simulink model "sampleModel646original"  (R2021b)
settings: Solver=VariableStepAuto  StartTime=0.0  StopTime=10.0  RelTol=1e-3
undefined symbols (not defined in the file): DiscIntNeverNeededParam, Newton, Raphson, sigbuilder_block
libraries: simulink x194, slpidlib x27
(part 1 of 5)
settings Model: Creator=user  LastModifiedBy=cemery

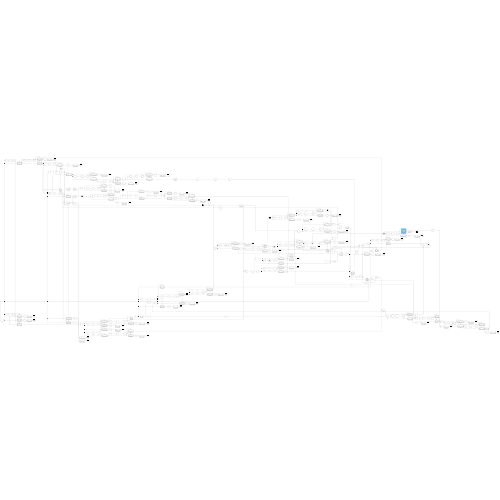
[thumbnail: Simulink's stored preview of the top-level diagram]
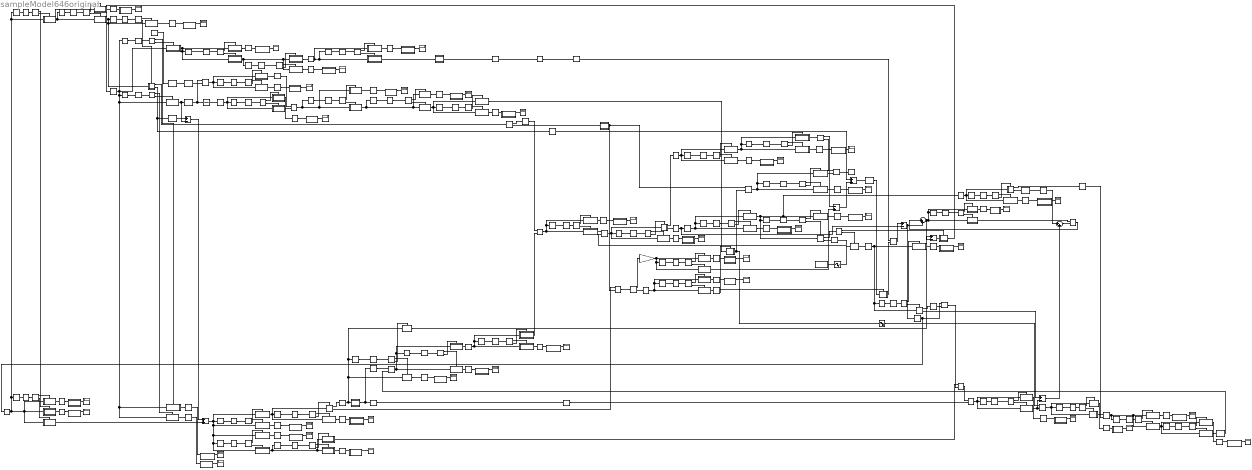
== system sampleModel646original ==
  cfblk1 : Delay  DelayLengthSource=Input port  SampleTime=1
      settings: InputPortMap=u0,p1
  cfblk10 : Subsystem  TreatAsAtomicUnit=on
  cfblk100 : Subsystem  TreatAsAtomicUnit=on
  cfblk101 : Subsystem  TreatAsAtomicUnit=on
  cfblk102 : Subsystem  TreatAsAtomicUnit=on
  cfblk{103..104,109..113} (7 alike) : Delay  SampleTime=1
  cfblk105 : Subsystem  TreatAsAtomicUnit=on
  cfblk106 : Subsystem  TreatAsAtomicUnit=on
  cfblk107 : Subsystem  TreatAsAtomicUnit=on
  cfblk108 : Subsystem  TreatAsAtomicUnit=on
  cfblk11 : Subsystem  TreatAsAtomicUnit=on
  cfblk12 : Subsystem  TreatAsAtomicUnit=on
  cfblk13 : Subsystem  TreatAsAtomicUnit=on
  cfblk14 : Product  Inputs=*
  cfblk15 : Gain  Gain=[-46724014.204909]
  cfblk16 : Sum
  cfblk17 : Subsystem  TreatAsAtomicUnit=on
  cfblk18 : Subsystem  TreatAsAtomicUnit=on
  cfblk19 : Subsystem  TreatAsAtomicUnit=on
  cfblk2 : simulink/Discrete/Tapped Delay  vinit=0.0  samptime=-1  NumDelays=1  DelayOrder=Oldest  includeCurrent=off
  cfblk20 : ComplexToMagnitudeAngle
  cfblk21 : PermuteDimensions
  cfblk22 : Sqrt  Operator=rSqrt  AlgorithmType=Newton-Raphson  SaturateOnIntegerOverflow=on
  cfblk23 : Reshape
  cfblk24 : Subsystem  TreatAsAtomicUnit=on
  cfblk25 : Subsystem  TreatAsAtomicUnit=on
  cfblk26 : Subsystem  TreatAsAtomicUnit=on
  cfblk27 : Subsystem  TreatAsAtomicUnit=on
  cfblk28 : Assignment  DiagnosticForDimensions=Warning  IndexOptions=Index vector (dialog)  Indices=1  OutputSizes=1
  cfblk29 : Sum
  cfblk3 : Subsystem  TreatAsAtomicUnit=on
  cfblk30 : Sqrt  SaturateOnIntegerOverflow=on
  cfblk31 : Squeeze
  cfblk32 : ComplexToMagnitudeAngle
  cfblk33 : Product  Inputs=**
  cfblk{34,49,60,72} (4 alike) : Sum  Inputs=+-
  cfblk35 : Subsystem  TreatAsAtomicUnit=on
  cfblk36 : Assignment  DiagnosticForDimensions=Warning  IndexOptions=Index vector (dialog)  Indices=1  OutputSizes=1
  cfblk37 : Subsystem  TreatAsAtomicUnit=on
  cfblk38 : Math  Operator=hermitian  SaturateOnIntegerOverflow=on
  cfblk39 : Math  Operator=pow  SaturateOnIntegerOverflow=on
  cfblk4 : DiscreteFilter  SampleTime=1
  cfblk40 : Subsystem  TreatAsAtomicUnit=on
  cfblk41 : simulink/Math Operations/MinMax Running Resettable  Function=min  vinit=0.0
  cfblk42 : Sqrt  Operator=rSqrt  AlgorithmType=Newton-Raphson  SaturateOnIntegerOverflow=on
  cfblk43 : DotProduct  InputSameDT=on  OutDataTypeStr=Inherit: Inherit via internal rule
  cfblk44 : PermuteDimensions
  cfblk45 : Subsystem  TreatAsAtomicUnit=on
  cfblk46 : simulink/Math Operations/Slider Gain  gain=1  low=0  high=2
  cfblk47 : Squeeze
  cfblk48 : simulink/Math Operations/MinMax Running Resettable  Function=min  vinit=0.0
  cfblk5 : Sum  Inputs=+
  cfblk50 : UnaryMinus
  cfblk51 : Subsystem  TreatAsAtomicUnit=on
  cfblk52 : Sin  TimeSource=Use external signal  SampleTime=0
  cfblk53 : Product
  cfblk54 : Subsystem  TreatAsAtomicUnit=on
  cfblk55 : Sum  Inputs=|++
  cfblk56 : Subsystem  TreatAsAtomicUnit=on
  cfblk57 : Sum  Inputs=|++
  cfblk58 : Product  Inputs=**
  cfblk59 : Subsystem  TreatAsAtomicUnit=on
  cfblk6 : Sin  TimeSource=Use external signal  SampleTime=0
  cfblk61 : Sum  Inputs=-+
  cfblk62 : Rounding
  cfblk63 : Product  Inputs=**
  cfblk64 : Polyval  Coefs=[ +2.081618890e-019, -1.441693666e-014, +4.719686976e-010, -8.536869453e-006, +1.621573104e-001, -8.087801117e+001 ]
  cfblk65 : DotProduct  InputSameDT=on  OutDataTypeStr=Inherit: Inherit via internal rule
  cfblk66 : Subsystem  TreatAsAtomicUnit=on
  cfblk67 : Subsystem  TreatAsAtomicUnit=on
  cfblk68 : ComplexToRealImag
  cfblk69 : Subsystem  TreatAsAtomicUnit=on
  cfblk7 : Sum  Inputs=+
  cfblk70 : Assignment  DiagnosticForDimensions=Warning  IndexOptions=Index vector (dialog)  Indices=1  OutputSizes=1
  cfblk71 : Subsystem  TreatAsAtomicUnit=on
  cfblk73 : Subsystem  TreatAsAtomicUnit=on
  cfblk74 : simulink/Math Operations/MinMax Running Resettable  Function=min  vinit=0.0
  cfblk75 : Signum
  cfblk76 : Product
  cfblk77 : Subsystem  TreatAsAtomicUnit=on
  cfblk78 : Subsystem  TreatAsAtomicUnit=on
  cfblk79 : Subsystem  TreatAsAtomicUnit=on
  cfblk8 : Polyval  Coefs=[ +2.081618890e-019, -1.441693666e-014, +4.719686976e-010, -8.536869453e-006, +1.621573104e-001, -8.087801117e+001 ]
  cfblk80 : Record  FileSettingsInternal="{\"entries\":[{\"content\":{\"excelSettings\":{\"content\":{},\"type\":\"Streamout.ExcelSettings\"}},\"type\":\"Streamout.FileSettingStorage\",\"uuid\":\"e31ca8c7-b91f-4ba9-b0e1-ad11411b0a50\"}],\"packageUris\":[\"http://schema.mathworks.com/mf0/streamout_blocks/R2020a\"],\"version\":\"1.0\"}"  SignalsInternal="{\"entries\":[{\"content\":{\"signals\":[{\"content\":{\"blockPath\":[\"sampleModel646original/cfblk80\"],\"channel\":[],\"dimensions\":[1],\"domain\":\"sampleModel646original/cfblk80\",\"lineColor\":\"#b746ff\",\"plots\":[1],\"port\":1,\"sid\":[],\"signalID\":136863,\"signalName\":\"cfblk28\"},\"type\":\"RecordBlkView.Signal\",\"uuid\":\"c95cab86-d875-48f3-a4b0-53c195fd7b48\"}]},\"type\":\"RecordBlkView.InputSignals\",\"uuid\":\"9f469ef3-1c0e-412c-9037-90f7de596239\"}],\"packageUris\":[\"http://schema.mathworks.com/mf0/streamout_blocks/R2020a\"],\"version\":\"1.0\"}"  VisualizationBindings="{\"sparklinesplugin\":{\"info\":[{\"bindingParametersList\":[],\"subplotID\":1}]}}"
  cfblk81 : UniformRandomNumber  Minimum=[-7025544522.327944]  Maximum=[7107108995.429539]  Seed=[76958620.000000]  SampleTime=0.1
  cfblk82 : Constant  Value=[557625621.134130]  SampleTime=1
  cfblk83 : Subsystem  TreatAsAtomicUnit=on
  cfblk84 : Subsystem
  cfblk85 : Subsystem
  cfblk86 : Subsystem
  cfblk87 : Subsystem
  cfblk88 : Subsystem
  cfblk89 : Subsystem
  cfblk9 : Subsystem  TreatAsAtomicUnit=on
  cfblk90 : Subsystem
  cfblk91 : Subsystem
  cfblk92 : Subsystem
  cfblk93 : Subsystem
  cfblk94 : If  IfExpression=u1 >= 0  SampleTime=1
  cfblk95 : If  IfExpression=u1 >= 0  SampleTime=1
  cfblk96 : Subsystem  TreatAsAtomicUnit=on
  cfblk97 : Subsystem  TreatAsAtomicUnit=on
  cfblk98 : Subsystem  TreatAsAtomicUnit=on
  cfblk99 : Subsystem  TreatAsAtomicUnit=on
  emi_{20,75,130,195,229,296,454,555,603,716,966,1015,1204,1372,1410,1493,1576,1865,1918,1992,2049} (21 alike) : Delay  SampleTime=1
  emi_{21,76,131,196,230,297,366,455,505,556,604,654,717,799,852,902,967,1016,1100,1147,1205,1297,1373,1411,1494,1577,1657,1751,1806,1866,1919,1993,2050,2123,2157,2192,2243} (37 alike) : Display
  emi_1017 : Subsystem
  emi_{462,574,619,690,760,832,912,976,1054,1118,1248,1338,1392,1441,1774,1888,1936,2012,2071,2136,2174,2204,2262} (23 alike) : If  IfExpression=0 > u1
  emi_{56,84,161,206,249,327,406,463,531,575,620,691,761,833,882,913,977,1055,1119,1163,1249,1339,1393,1442,1522,1609,1695,1775,1837,1889,1937,2013,2072,2137,2175,2205,2263} (37 alike) : DataTypeConversion  OutDataTypeStr=double
  emi_{85,207,250,407,464,576,621,762,834,978,1056,1120,1250,1340,1394,1443,1696,1776,1890,1938,2073,2138,2176,2206,2264} (25 alike) : Delay  InitialCondition=0
  emi_1061 : Subsystem  TreatAsAtomicUnit=on
  emi_{365,504,653,798,851,901,1099,1146,1296,1656,1750,1805,2122,2156,2191,2242} (16 alike) : Delay
  emi_1101 : Subsystem
  emi_1124 : Subsystem  TreatAsAtomicUnit=on
  emi_1148 : Subsystem
  emi_1162 : If  IfExpression=-1.382844e+09 > u1
  emi_1164 : Delay  InitialCondition=-691422001.6653
  emi_1168 : Subsystem  TreatAsAtomicUnit=on
  emi_1206 : Subsystem
  emi_1254 : Subsystem  TreatAsAtomicUnit=on
  emi_1298 : Subsystem
  emi_132 : Subsystem
  emi_1344 : Subsystem  TreatAsAtomicUnit=on
  emi_1374 : Subsystem
  emi_1399 : Subsystem  TreatAsAtomicUnit=on
  emi_1412 : Subsystem
  emi_1447 : Subsystem  TreatAsAtomicUnit=on
  emi_1495 : Subsystem
  emi_{530,881,1521,1608} (4 alike) : If  IfExpression=-1.617560e+02 > u1
  emi_{328,532,883,1523,1610} (5 alike) : Delay  InitialCondition=-80.878
  emi_1527 : Subsystem  TreatAsAtomicUnit=on
  emi_1578 : Subsystem
  emi_{83,160,205,248,1694} (5 alike) : If  IfExpression=0 > u1  SampleTime=1
  emi_1614 : Subsystem  TreatAsAtomicUnit=on
  emi_162 : Delay  InitialCondition=1
  emi_1658 : Subsystem
  emi_166 : Subsystem  TreatAsAtomicUnit=on
  emi_1700 : Subsystem  TreatAsAtomicUnit=on
  emi_1752 : Subsystem
  emi_1781 : Subsystem  TreatAsAtomicUnit=on
  emi_1807 : Subsystem
  emi_1836 : If  IfExpression=-2 > u1
  emi_1838 : Delay  InitialCondition=-1
  emi_1842 : Subsystem  TreatAsAtomicUnit=on
  emi_1867 : Subsystem
  emi_1894 : Subsystem  TreatAsAtomicUnit=on
  emi_1920 : Subsystem
  emi_1942 : Subsystem  TreatAsAtomicUnit=on
  emi_197 : Subsystem
  emi_1994 : Subsystem
  emi_2014 : Delay  InitialCondition=1.0441
  emi_2018 : Subsystem  TreatAsAtomicUnit=on
  emi_2051 : Subsystem
  emi_2077 : Subsystem  TreatAsAtomicUnit=on
  emi_211 : Subsystem  TreatAsAtomicUnit=on
  emi_2124 : Subsystem
  emi_2143 : Subsystem  TreatAsAtomicUnit=on
  emi_2158 : Subsystem
  emi_2180 : Subsystem  TreatAsAtomicUnit=on
  emi_2193 : Subsystem
  emi_22 : Subsystem
  emi_2210 : Subsystem  TreatAsAtomicUnit=on
  emi_2244 : Subsystem
  emi_231 : Subsystem
  emi_254 : Subsystem  TreatAsAtomicUnit=on
  emi_298 : Subsystem
  emi_3 : Subsystem  TreatAsAtomicUnit=on
  emi_326 : If  IfExpression=-1.617560e+02 > u1  SampleTime=1
  emi_332 : Subsystem  TreatAsAtomicUnit=on
  emi_367 : Subsystem
  emi_405 : If  IfExpression=0 > u1  SampleTime=0
  emi_411 : Subsystem  TreatAsAtomicUnit=on
  emi_456 : Subsystem
  emi_468 : Subsystem  TreatAsAtomicUnit=on
  emi_506 : Subsystem
  emi_536 : Subsystem  TreatAsAtomicUnit=on
  emi_55 : If  IfExpression=-1.382844e+09 > u1  SampleTime=1
  emi_557 : Subsystem
  emi_57 : Delay  InitialCondition=-691422001.6653
  emi_580 : Subsystem  TreatAsAtomicUnit=on
  emi_605 : Subsystem
  emi_61 : Subsystem  TreatAsAtomicUnit=on
  emi_625 : Subsystem  TreatAsAtomicUnit=on
  emi_655 : Subsystem
  emi_692 : Delay  InitialCondition=80.878
  emi_697 : Subsystem  TreatAsAtomicUnit=on
  emi_718 : Subsystem
  emi_766 : Subsystem  TreatAsAtomicUnit=on
  emi_77 : Subsystem
  emi_800 : Subsystem
  emi_838 : Subsystem  TreatAsAtomicUnit=on
  emi_853 : Subsystem
  emi_888 : Subsystem  TreatAsAtomicUnit=on
  emi_89 : Subsystem  TreatAsAtomicUnit=on
  emi_903 : Subsystem
  emi_914 : Delay  InitialCondition=56986100045.4225
  emi_918 : Subsystem  TreatAsAtomicUnit=on
  emi_968 : Subsystem
  emi_982 : Subsystem  TreatAsAtomicUnit=on
  wires:
  emi_248/1 -> emi_211/Action
  emi_2264/1 -> emi_2263/1
  emi_2263/1 -> emi_2262/1
  emi_207/1 -> emi_206/1
  emi_2242/1 -> emi_2244/1(In1)
  emi_2262/1 -> emi_2210/Action
  emi_2210/1(emi_2218) -> emi_2242/1
  emi_2180/1(emi_2188) -> emi_2191/1
  emi_2191/1 -> emi_2193/1(In1)
  emi_2262/2 -> cfblk37/Action
  emi_1918/1 -> emi_1920/1(In1)
  cfblk93/1(cfblk2) -> cfblk38/1
  emi_760/2 -> cfblk18/Action
  emi_2204/2 -> cfblk83/Action
  emi_761/1 -> emi_760/1
  emi_2244/1(Out1) -> emi_2243/1
  emi_2156/1 -> emi_2158/1(In1)
  cfblk37/1(emi_2209) -> cfblk42/1
  cfblk101/1(emi_60) -> cfblk39/1
  emi_2206/1 -> emi_2205/1
  emi_1163/1 -> emi_1162/1
  emi_2205/1 -> emi_2204/1
  emi_2204/1 -> emi_2180/Action
  emi_2193/1(Out1) -> emi_2192/1
  cfblk19/2(emi_2142) -> cfblk49/1
  cfblk83/1(emi_2179) -> cfblk90/1(cfblk1)
  cfblk105/1(emi_88) -> cfblk72/1
  emi_2176/1 -> emi_2175/1
  emi_2122/1 -> emi_2124/1(In1)
  emi_2175/1 -> emi_2174/1
  emi_2072/1 -> emi_2071/1
  emi_130/1 -> emi_132/1(In1)
  emi_2174/2 -> cfblk19/Action
  cfblk88/1(cfblk2) -> cfblk74/2, cfblk53/1
  emi_2174/1 -> emi_2143/Action
  emi_1392/2 -> cfblk54/Action
  emi_2158/1(Out1) -> emi_2157/1
  emi_2077/1(emi_2085) -> emi_2122/1
  emi_2143/1(emi_2151) -> emi_2156/1
  emi_977/1 -> emi_976/1
  emi_1888/2 -> cfblk77/Action
  cfblk22/1 -> cfblk41/2
  emi_976/1 -> emi_918/Action
  emi_1890/1 -> emi_1889/1
  emi_365/1 -> emi_367/1(In1)
  emi_1938/1 -> emi_1937/1
  emi_766/1(emi_774) -> emi_798/1
  cfblk19/1(emi_2141) -> cfblk22/1
  emi_1920/1(Out1) -> emi_1919/1
  emi_2138/1 -> emi_2137/1
  emi_1992/1 -> emi_1994/1(In1)
  emi_1118/1 -> emi_1061/Action
  emi_1994/1(Out1) -> emi_1993/1
  emi_2071/2 -> cfblk9/Action
  emi_2137/1 -> emi_2136/1
  emi_2124/1(Out1) -> emi_2123/1
  emi_2136/1 -> emi_2077/Action
  emi_2136/2 -> cfblk10/Action
  cfblk10/1(emi_2076) -> cfblk32/1
  emi_2071/1 -> emi_2018/Action
  emi_2073/1 -> emi_2072/1
  emi_2049/1 -> emi_2051/1(In1)
  emi_2051/1(Out1) -> emi_2050/1
  emi_1936/1 -> emi_1894/Action
  cfblk95/1 -> cfblk98/Action
  emi_2018/1(emi_2026) -> emi_2049/1
  cfblk78/1(emi_1893) -> cfblk43/2
  cfblk9/1(emi_2017) -> cfblk28/2
  emi_2013/1 -> emi_2012/1
  emi_2014/1 -> emi_2013/1
  emi_2012/1 -> emi_1942/Action
  emi_1942/1(emi_1950) -> emi_1992/1
  emi_2012/2 -> cfblk79/Action
  emi_1867/1(Out1) -> emi_1866/1
  emi_1937/1 -> emi_1936/1
  emi_55/2 -> cfblk100/Action
  cfblk79/1(emi_1941) -> cfblk93/1(cfblk1)
  emi_56/1 -> emi_55/1
  emi_1894/1(emi_1902) -> emi_1918/1
  emi_77/1(Out1) -> emi_76/1
  emi_1936/2 -> cfblk78/Action
  cfblk89/1(cfblk2) -> cfblk5/1
  cfblk26/1(emi_886) -> cfblk20/1
  emi_1888/1 -> emi_1842/Action
  cfblk31/1 -> cfblk41/1, cfblk64/1
  emi_1889/1 -> emi_1888/1
  emi_1865/1 -> emi_1867/1(In1)
  emi_1842/1(emi_1850) -> emi_1865/1
  emi_1442/1 -> emi_1441/1
  emi_1838/1 -> emi_1837/1
  emi_1146/1 -> emi_1148/1(In1)
  emi_1837/1 -> emi_1836/1
  emi_1836/1 -> emi_1781/Action
  emi_1836/2 -> cfblk71/Action
  emi_1807/1(Out1) -> emi_1806/1
  emi_1805/1 -> emi_1807/1(In1)
  emi_132/1(Out1) -> emi_131/1
  emi_1781/1(emi_1789) -> emi_1805/1
  cfblk21/1 -> cfblk35/1(emi_1058), emi_1061/1(emi_1068), emi_1120/1
  cfblk71/2(emi_1780) -> cfblk74/1
  cfblk71/1(emi_1779) -> cfblk62/1
  cfblk74/1 -> cfblk68/1
  emi_1776/1 -> emi_1775/1
  emi_1775/1 -> emi_1774/1
  emi_1774/1 -> emi_1700/Action
  emi_57/1 -> emi_56/1
  emi_1774/2 -> cfblk73/Action
  emi_1162/1 -> emi_1124/Action
  emi_1752/1(Out1) -> emi_1751/1
  emi_1750/1 -> emi_1752/1(In1)
  emi_1700/1(emi_1708) -> emi_1750/1
  emi_1696/1 -> emi_1695/1
  emi_1695/1 -> emi_1694/1
  emi_1694/1 -> emi_1614/Action
  emi_1694/2 -> cfblk102/Action
  cfblk30/1 -> emi_211/1(emi_218), emi_250/1, cfblk107/1(emi_209)
  cfblk82/1 -> cfblk52/1
  emi_1658/1(Out1) -> emi_1657/1
  emi_1656/1 -> emi_1658/1(In1)
  emi_1614/1(emi_1622) -> emi_1656/1
  cfblk50/1 -> cfblk44/1, cfblk60/2
  cfblk102/1(emi_1613) -> cfblk99/1(cfblk1)
  emi_1610/1 -> emi_1609/1
  emi_1609/1 -> emi_1608/1
  emi_1608/1 -> emi_1527/Action
  emi_1608/2 -> cfblk66/Action
  emi_1578/1(Out1) -> emi_1577/1
  emi_506/1(Out1) -> emi_505/1
  emi_1576/1 -> emi_1578/1(In1)
  emi_468/1(emi_476) -> emi_504/1
  emi_1527/1(emi_1535) -> emi_1576/1
  emi_1523/1 -> emi_1522/1
  emi_454/1 -> emi_456/1(In1)
  emi_1522/1 -> emi_1521/1
  emi_1521/1 -> emi_1447/Action
  cfblk5/1 -> cfblk55/1
  emi_1521/2 -> cfblk59/Action
  emi_1495/1(Out1) -> emi_1494/1
  emi_1493/1 -> emi_1495/1(In1)
  emi_1447/1(emi_1455) -> emi_1493/1
  emi_1443/1 -> emi_1442/1
  emi_1441/1 -> emi_1399/Action
  emi_1441/2 -> cfblk56/Action
  emi_1162/2 -> cfblk40/Action
  emi_1412/1(Out1) -> emi_1411/1
  emi_1410/1 -> emi_1412/1(In1)
  emi_1399/1(emi_1407) -> emi_1410/1
  cfblk56/2(emi_1398) -> cfblk112/1
  cfblk56/1(emi_1397) -> cfblk94/1
  emi_1394/1 -> emi_1393/1
  emi_1393/1 -> emi_1392/1
  emi_1392/1 -> emi_1344/Action
  emi_1374/1(Out1) -> emi_1373/1
  emi_966/1 -> emi_968/1(In1)
  emi_1372/1 -> emi_1374/1(In1)
  emi_1344/1(emi_1352) -> emi_1372/1
  cfblk54/1(emi_1343) -> cfblk33/1
  emi_1340/1 -> emi_1339/1
  emi_1339/1 -> emi_1338/1
  emi_1338/1 -> emi_1254/Action
  emi_1338/2 -> cfblk69/Action
  emi_1298/1(Out1) -> emi_1297/1
  emi_1296/1 -> emi_1298/1(In1)
  emi_1254/1(emi_1262) -> emi_1296/1
  emi_55/1 -> emi_3/Action
  emi_1250/1 -> emi_1249/1
  emi_1249/1 -> emi_1248/1
  emi_1248/1 -> emi_1168/Action
  cfblk85/1(cfblk2) -> cfblk46/1, cfblk103/1
  emi_1248/2 -> cfblk51/Action
  emi_1206/1(Out1) -> emi_1205/1
  emi_367/1(Out1) -> emi_366/1
  emi_1204/1 -> emi_1206/1(In1)
  emi_1168/1(emi_1176) -> emi_1204/1
  emi_1164/1 -> emi_1163/1
  emi_575/1 -> emi_574/1
  emi_1148/1(Out1) -> emi_1147/1
  emi_1124/1(emi_1132) -> emi_1146/1
  emi_1120/1 -> emi_1119/1
  emi_1119/1 -> emi_1118/1
  emi_1118/2 -> cfblk35/Action
  cfblk111/1 -> cfblk16/1
  emi_1101/1(Out1) -> emi_1100/1
  emi_1099/1 -> emi_1101/1(In1)
  emi_1061/1(emi_1069) -> emi_1099/1
  cfblk36/1 -> cfblk100/1(emi_1), emi_3/1(emi_10), emi_57/1
  emi_576/1 -> emi_575/1
  cfblk35/2(emi_1060) -> cfblk89/1(cfblk1)
  cfblk35/1(emi_1059) -> cfblk113/1
  emi_1056/1 -> emi_1055/1
  cfblk46/1 -> cfblk104/1
  emi_1055/1 -> emi_1054/1
  emi_1054/1 -> emi_982/Action
  emi_1054/2 -> cfblk3/Action
  emi_1017/1(Out1) -> emi_1016/1
  emi_1015/1 -> emi_1017/1(In1)
  emi_982/1(emi_990) -> emi_1015/1
  cfblk72/1 -> cfblk96/1(cfblk1)
  cfblk3/1(emi_981) -> cfblk7/1
  emi_978/1 -> emi_977/1
  emi_976/2 -> cfblk27/Action
  emi_160/2 -> cfblk105/Action
  emi_968/1(Out1) -> emi_967/1
  emi_918/1(emi_926) -> emi_966/1
  emi_914/1 -> emi_913/1
  emi_913/1 -> emi_912/1
  emi_532/1 -> emi_531/1
  emi_912/1 -> emi_888/Action
  emi_557/1(Out1) -> emi_556/1
  emi_912/2 -> cfblk26/Action
  emi_555/1 -> emi_557/1(In1)
  emi_903/1(Out1) -> emi_902/1
  emi_901/1 -> emi_903/1(In1)
  emi_888/1(emi_896) -> emi_901/1
  emi_883/1 -> emi_882/1
  emi_882/1 -> emi_881/1
  emi_716/1 -> emi_718/1(In1)
  emi_881/1 -> emi_838/Action
  emi_881/2 -> cfblk25/Action
  emi_853/1(Out1) -> emi_852/1
  emi_851/1 -> emi_853/1(In1)
  emi_838/1(emi_846) -> emi_851/1
  cfblk25/1(emi_837) -> cfblk29/2
  emi_834/1 -> emi_833/1
  emi_833/1 -> emi_832/1
  cfblk60/1 -> cfblk31/1, cfblk57/2
  emi_832/1 -> emi_766/Action
  emi_832/2 -> cfblk24/Action
  emi_800/1(Out1) -> emi_799/1
  emi_798/1 -> emi_800/1(In1)
  emi_762/1 -> emi_761/1
  emi_760/1 -> emi_697/Action
  emi_718/1(Out1) -> emi_717/1
  emi_697/1(emi_705) -> emi_716/1
  cfblk48/1 -> cfblk60/1
  cfblk18/2(emi_696) -> cfblk50/1
  cfblk18/1(emi_695) -> cfblk14/1
  emi_692/1 -> emi_691/1
  cfblk32/1 -> cfblk61/1
  emi_691/1 -> emi_690/1
  emi_690/1 -> emi_625/Action
  emi_690/2 -> cfblk17/Action
  emi_655/1(Out1) -> emi_654/1
  emi_653/1 -> emi_655/1(In1)
  emi_603/1 -> emi_605/1(In1)
  emi_625/1(emi_633) -> emi_653/1
  emi_621/1 -> emi_620/1
  emi_620/1 -> emi_619/1
  emi_619/1 -> emi_580/Action
  emi_619/2 -> cfblk13/Action
  cfblk75/1 -> emi_918/1(emi_925), emi_1168/1(emi_1175), cfblk27/1(emi_916), emi_978/1, cfblk51/1(emi_1166), emi_1250/1
  emi_605/1(Out1) -> emi_604/1
  emi_580/1(emi_588) -> emi_603/1
  cfblk13/1(emi_579) -> cfblk8/1
  emi_574/1 -> emi_536/Action
  emi_574/2 -> cfblk67/Action
  emi_326/2 -> cfblk108/Action
  emi_536/1(emi_544) -> emi_555/1
  emi_531/1 -> emi_530/1
  emi_530/1 -> emi_468/Action
  emi_530/2 -> cfblk12/Action
  emi_504/1 -> emi_506/1(In1)
  emi_464/1 -> emi_463/1
  emi_463/1 -> emi_462/1
  emi_462/1 -> emi_411/Action
  emi_462/2 -> cfblk11/Action
  emi_456/1(Out1) -> emi_455/1
  emi_411/1(emi_419) -> emi_454/1
  emi_407/1 -> emi_406/1
  emi_406/1 -> emi_405/1
  emi_405/1 -> emi_332/Action
  emi_405/2 -> cfblk45/Action
  emi_332/1(emi_340) -> emi_365/1
  cfblk45/1(emi_331) -> cfblk70/2
  emi_328/1 -> emi_327/1
  emi_327/1 -> emi_326/1
  emi_326/1 -> emi_254/Action
  emi_298/1(Out1) -> emi_297/1
  emi_296/1 -> emi_298/1(In1)
  emi_254/1(emi_262) -> emi_296/1
  cfblk108/1(emi_253) -> cfblk63/1
  emi_250/1 -> emi_249/1
  emi_249/1 -> emi_248/1
  emi_248/2 -> cfblk107/Action
  emi_231/1(Out1) -> emi_230/1
  emi_229/1 -> emi_231/1(In1)
  emi_211/1(emi_219) -> emi_229/1
  cfblk107/1(emi_210) -> cfblk95/1
  emi_206/1 -> emi_205/1
  emi_205/1 -> emi_166/Action
  emi_205/2 -> cfblk106/Action
  emi_197/1(Out1) -> emi_196/1
  emi_195/1 -> emi_197/1(In1)
  emi_166/1(emi_174) -> emi_195/1
  cfblk43/1 -> emi_1394/1, emi_1344/1(emi_1351), cfblk54/1(emi_1342)
  cfblk106/1(emi_165) -> cfblk61/2
  emi_162/1 -> emi_161/1
  emi_161/1 -> emi_160/1
  cfblk92/1(cfblk2) -> cfblk98/1(cfblk1)
  emi_160/1 -> emi_89/Action
  cfblk11/1(emi_410) -> cfblk49/2, cfblk36/2
  emi_89/1(emi_97) -> emi_130/1
  cfblk40/1(emi_1123) -> cfblk83/1(emi_2178), emi_2180/1(emi_2187), emi_2206/1
  emi_85/1 -> emi_84/1
  emi_84/1 -> emi_83/1
  emi_83/1 -> emi_61/Action
  emi_83/2 -> cfblk101/Action
  emi_75/1 -> emi_77/1(In1)
  cfblk24/1(emi_765) -> cfblk102/1(emi_1612), emi_1614/1(emi_1621), emi_1696/1
  emi_61/1(emi_69) -> emi_75/1
  emi_22/1(Out1) -> emi_21/1
  cfblk94/2 -> cfblk97/Action
  emi_20/1 -> emi_22/1(In1)
  emi_3/1(emi_11) -> emi_20/1
  cfblk100/1(emi_2) -> cfblk1/1
  cfblk113/1 -> cfblk1/2
  cfblk112/1 -> cfblk33/2
  cfblk110/1 -> cfblk43/1
  cfblk20/1 -> cfblk110/1
  cfblk109/1 -> cfblk48/1
  cfblk47/1 -> cfblk109/1
  cfblk104/1 -> cfblk58/2
  cfblk103/1 -> cfblk65/1
  cfblk95/2 -> cfblk99/Action
  cfblk94/1 -> cfblk96/Action
  cfblk65/1 -> cfblk3/1(emi_980), emi_1056/1, emi_982/1(emi_989)
  cfblk90/1(cfblk2) -> cfblk65/2
  cfblk49/1 -> cfblk55/2
  cfblk87/1(cfblk2) -> cfblk34/1
  cfblk16/1 -> cfblk92/1(cfblk1)
  cfblk39/1 -> cfblk57/1
  cfblk41/1 -> cfblk63/2
  cfblk38/1 -> cfblk47/1
  cfblk28/1 -> cfblk80/1
  cfblk91/1(cfblk2) -> cfblk76/2
  cfblk4/1 -> cfblk23/1
  cfblk32/2 -> cfblk28/1
  cfblk81/1 -> cfblk84/1(cfblk1)
  cfblk6/1 -> cfblk36/1
  cfblk61/1 -> cfblk16/2
  cfblk20/2 -> cfblk88/1(cfblk1)
  cfblk55/1 -> cfblk39/2
  cfblk96/1(cfblk2) -> cfblk75/1
  cfblk76/1 -> cfblk13/1(emi_578), emi_580/1(emi_587), emi_621/1
  cfblk84/1(cfblk2) -> cfblk91/1(cfblk1)
  cfblk34/1 -> cfblk29/1
  cfblk97/1(cfblk2) -> cfblk2/1
  cfblk52/1 -> cfblk97/1(cfblk1)
  cfblk68/2 -> cfblk30/1
  cfblk68/1 -> cfblk15/1
  cfblk67/1(emi_535) -> cfblk24/1(emi_764), emi_766/1(emi_773), emi_834/1
  cfblk98/1(cfblk2) -> cfblk48/2
  cfblk63/1 -> cfblk58/1
  cfblk8/1 -> cfblk70/1
  cfblk69/1(emi_1253) -> cfblk37/1(emi_2208), emi_2210/1(emi_2217), emi_2264/1
  cfblk1/1 -> cfblk40/1(emi_1122), emi_1124/1(emi_1131), emi_1164/1
  cfblk2/1 -> cfblk19/1(emi_2140), emi_2176/1, emi_2143/1(emi_2150)
  cfblk77/1(emi_1841) -> cfblk10/1(emi_2075), emi_2138/1, emi_2077/1(emi_2084)
  cfblk53/1 -> cfblk9/1(emi_2016), emi_2073/1, emi_2018/1(emi_2025)
  cfblk42/1 -> cfblk79/1(emi_1940), emi_2014/1, emi_1942/1(emi_1949)
  cfblk7/1 -> cfblk78/1(emi_1892), emi_1938/1, emi_1894/1(emi_1901)
  cfblk14/1 -> cfblk77/1(emi_1840), emi_1842/1(emi_1849), emi_1890/1
  cfblk59/1(emi_1446) -> cfblk71/1(emi_1778), emi_1781/1(emi_1788), emi_1838/1
  cfblk33/1 -> cfblk18/1(emi_694), emi_697/1(emi_704), emi_762/1
  cfblk73/1(emi_1699) -> cfblk56/1(emi_1396), emi_1443/1, emi_1399/1(emi_1406), cfblk21/1
  cfblk44/1 -> cfblk73/1(emi_1698), emi_1776/1, emi_1700/1(emi_1707)
  cfblk66/1(emi_1526) -> emi_254/1(emi_261), cfblk108/1(emi_252), emi_328/1
  cfblk51/1(emi_1167) -> cfblk69/1(emi_1252), emi_1340/1, emi_1254/1(emi_1261)
  cfblk27/1(emi_917) -> cfblk34/2, cfblk86/1(cfblk1)
  cfblk26/2(emi_887) -> cfblk111/1, cfblk87/1(cfblk1)
  cfblk17/1(emi_624) -> cfblk26/1(emi_885), emi_888/1(emi_895), emi_914/1
  cfblk12/1(emi_467) -> cfblk17/1(emi_623), emi_692/1, emi_625/1(emi_632)
  cfblk70/1 -> cfblk67/1(emi_534), emi_536/1(emi_543), emi_576/1
  cfblk58/1 -> cfblk11/1(emi_409), emi_411/1(emi_418), emi_464/1
  cfblk23/1 -> cfblk45/1(emi_330), emi_332/1(emi_339), emi_407/1
  cfblk15/1 -> cfblk106/1(emi_164), emi_207/1, emi_166/1(emi_173)
  cfblk62/1 -> cfblk105/1(emi_87), emi_162/1, emi_89/1(emi_96), cfblk85/1(cfblk1)
  cfblk86/1(cfblk2) -> cfblk76/1, cfblk4/1
  cfblk57/1 -> emi_61/1(emi_68), emi_85/1, cfblk101/1(emi_59), cfblk72/2
  cfblk99/1(cfblk2) -> cfblk6/1, cfblk53/2
  cfblk29/1 -> emi_1610/1, cfblk66/1(emi_1525), emi_1527/1(emi_1534), emi_1447/1(emi_1454), emi_1523/1, cfblk59/1(emi_1445)
  cfblk64/1 -> cfblk25/1(emi_836), emi_838/1(emi_845), emi_468/1(emi_475), emi_532/1, cfblk12/1(emi_466), emi_883/1

== system sampleModel646original/cfblk10 ==
  emi_2075 : Inport
  Action Port : ActionPort  ActionPortLabel=else
  cfblk10 : Reshape
  emi_2076 : Outport
  wires:
  emi_2075/1 -> cfblk10/1
  cfblk10/1 -> emi_2076/1

== system sampleModel646original/cfblk100 ==
  emi_1 : Inport
  Action Port : ActionPort  ActionPortLabel=else
  cfblk100 : Delay  SampleTime=1
  emi_2 : Outport
  wires:
  emi_1/1 -> cfblk100/1
  cfblk100/1 -> emi_2/1

== system sampleModel646original/cfblk101 ==
  emi_59 : Inport
  Action Port : ActionPort  ActionPortLabel=else
  cfblk101 : Delay  SampleTime=1
  emi_60 : Outport
  wires:
  emi_59/1 -> cfblk101/1
  cfblk101/1 -> emi_60/1

== system sampleModel646original/cfblk102 ==
  emi_1612 : Inport
  Action Port : ActionPort  ActionPortLabel=else
  cfblk102 : Delay  SampleTime=1
  emi_1613 : Outport
  wires:
  emi_1612/1 -> cfblk102/1
  cfblk102/1 -> emi_1613/1

== system sampleModel646original/cfblk105 ==
  emi_87 : Inport
  Action Port : ActionPort  ActionPortLabel=else
  cfblk105 : Delay  SampleTime=1
  emi_88 : Outport
  wires:
  emi_87/1 -> cfblk105/1
  cfblk105/1 -> emi_88/1

== system sampleModel646original/cfblk106 ==
  emi_164 : Inport
  Action Port : ActionPort  ActionPortLabel=else
  cfblk106 : Delay  SampleTime=1
  emi_165 : Outport
  wires:
  emi_164/1 -> cfblk106/1
  cfblk106/1 -> emi_165/1

== system sampleModel646original/cfblk107 ==
  emi_209 : Inport
  Action Port : ActionPort  ActionPortLabel=else
  cfblk107 : Delay  SampleTime=1
  emi_210 : Outport
  wires:
  emi_209/1 -> cfblk107/1
  cfblk107/1 -> emi_210/1

== system sampleModel646original/cfblk108 ==
  emi_252 : Inport
  Action Port : ActionPort  ActionPortLabel=else
  cfblk108 : Delay  SampleTime=1
  emi_253 : Outport
  wires:
  emi_252/1 -> cfblk108/1
  cfblk108/1 -> emi_253/1

== system sampleModel646original/cfblk11 ==
  emi_409 : Inport
  Action Port : ActionPort  ActionPortLabel=else
  cfblk11 : Bias  Bias=[-691422001.665259]
  emi_410 : Outport
  wires:
  emi_409/1 -> cfblk11/1
  cfblk11/1 -> emi_410/1

== system sampleModel646original/cfblk12 ==
  emi_466 : Inport
  Action Port : ActionPort  ActionPortLabel=else
  cfblk12 : Abs
  emi_467 : Outport
  wires:
  emi_466/1 -> cfblk12/1
  cfblk12/1 -> emi_467/1

== system sampleModel646original/cfblk13 ==
  emi_578 : Inport
  Action Port : ActionPort  ActionPortLabel=else
  cfblk13 : Trigonometry
  emi_579 : Outport
  wires:
  emi_578/1 -> cfblk13/1
  cfblk13/1 -> emi_579/1

== system sampleModel646original/cfblk17 ==
  emi_623 : Inport
  Action Port : ActionPort  ActionPortLabel=else
  cfblk17 : Gain  Gain=[704593241.364970]
  emi_624 : Outport
  wires:
  emi_623/1 -> cfblk17/1
  cfblk17/1 -> emi_624/1

== system sampleModel646original/cfblk18 ==
  emi_694 : Inport
  Action Port : ActionPort  ActionPortLabel=else
  cfblk18 : ComplexToMagnitudeAngle
  emi_695 : Outport
  emi_696 : Outport  Port=2
  wires:
  emi_694/1 -> cfblk18/1
  cfblk18/1 -> emi_695/1
  cfblk18/2 -> emi_696/1

== system sampleModel646original/cfblk19 ==
  emi_2140 : Inport
  Action Port : ActionPort  ActionPortLabel=else
  cfblk19 : ComplexToMagnitudeAngle
  emi_2141 : Outport
  emi_2142 : Outport  Port=2
  wires:
  emi_2140/1 -> cfblk19/1
  cfblk19/1 -> emi_2141/1
  cfblk19/2 -> emi_2142/1

== system sampleModel646original/cfblk24 ==
  emi_764 : Inport
  Action Port : ActionPort  ActionPortLabel=else
  cfblk24 : UnaryMinus
  emi_765 : Outport
  wires:
  emi_764/1 -> cfblk24/1
  cfblk24/1 -> emi_765/1

== system sampleModel646original/cfblk25 ==
  emi_836 : Inport
  Action Port : ActionPort  ActionPortLabel=else
  cfblk25 : Product  Inputs=*
  emi_837 : Outport
  wires:
  emi_836/1 -> cfblk25/1
  cfblk25/1 -> emi_837/1

== system sampleModel646original/cfblk26 ==
  emi_885 : Inport
  Action Port : ActionPort  ActionPortLabel=else
  cfblk26 : ComplexToMagnitudeAngle
  emi_886 : Outport
  emi_887 : Outport  Port=2
  wires:
  emi_885/1 -> cfblk26/1
  cfblk26/1 -> emi_886/1
  cfblk26/2 -> emi_887/1

== system sampleModel646original/cfblk27 ==
  emi_916 : Inport
  Action Port : ActionPort  ActionPortLabel=else
  cfblk27 : Gain  Gain=[-262585566.335352]
  emi_917 : Outport
  wires:
  emi_916/1 -> cfblk27/1
  cfblk27/1 -> emi_917/1

== system sampleModel646original/cfblk3 ==
  emi_980 : Inport
  Action Port : ActionPort  ActionPortLabel=else
  cfblk3 : simulink/Discrete/Transfer Fcn First Order  PoleZ=0.95  ICPrevOutput=0.0  DoSatur=off
  emi_981 : Outport
  wires:
  emi_980/1 -> cfblk3/1
  cfblk3/1 -> emi_981/1

== system sampleModel646original/cfblk35 ==
  emi_1058 : Inport
  Action Port : ActionPort  ActionPortLabel=else
  cfblk35 : ComplexToMagnitudeAngle
  emi_1059 : Outport
  emi_1060 : Outport  Port=2
  wires:
  emi_1058/1 -> cfblk35/1
  cfblk35/1 -> emi_1059/1
  cfblk35/2 -> emi_1060/1

== system sampleModel646original/cfblk37 ==
  emi_2208 : Inport
  Action Port : ActionPort  ActionPortLabel=else
  cfblk37 : Sum  Inputs=+
  emi_2209 : Outport
  wires:
  emi_2208/1 -> cfblk37/1
  cfblk37/1 -> emi_2209/1

== system sampleModel646original/cfblk40 ==
  emi_1122 : Inport
  Action Port : ActionPort  ActionPortLabel=else
  cfblk40 : Gain  Gain=[-69220576.399279]
  emi_1123 : Outport
  wires:
  emi_1122/1 -> cfblk40/1
  cfblk40/1 -> emi_1123/1

== system sampleModel646original/cfblk45 ==
  emi_330 : Inport
  Action Port : ActionPort  ActionPortLabel=else
  cfblk45 : Sin  TimeSource=Use external signal  SampleTime=0
  emi_331 : Outport
  wires:
  emi_330/1 -> cfblk45/1
  cfblk45/1 -> emi_331/1

== system sampleModel646original/cfblk51 ==
  emi_1166 : Inport
  Action Port : ActionPort  ActionPortLabel=else
  cfblk51 : Trigonometry
  emi_1167 : Outport
  wires:
  emi_1166/1 -> cfblk51/1
  cfblk51/1 -> emi_1167/1

== system sampleModel646original/cfblk54 ==
  emi_1342 : Inport
  Action Port : ActionPort  ActionPortLabel=else
  cfblk54 : Reshape
  emi_1343 : Outport
  wires:
  emi_1342/1 -> cfblk54/1
  cfblk54/1 -> emi_1343/1

== system sampleModel646original/cfblk56 ==
  emi_1396 : Inport
  Action Port : ActionPort  ActionPortLabel=else
  cfblk56 : ComplexToRealImag
  emi_1397 : Outport
  emi_1398 : Outport  Port=2
  wires:
  emi_1396/1 -> cfblk56/1
  cfblk56/1 -> emi_1397/1
  cfblk56/2 -> emi_1398/1

== system sampleModel646original/cfblk59 ==
  emi_1445 : Inport
  Action Port : ActionPort  ActionPortLabel=else
  cfblk59 : Signum
  emi_1446 : Outport
  wires:
  emi_1445/1 -> cfblk59/1
  cfblk59/1 -> emi_1446/1

== system sampleModel646original/cfblk66 ==
  emi_1525 : Inport
  Action Port : ActionPort  ActionPortLabel=else
  cfblk66 : Product  Inputs=*
  emi_1526 : Outport
  wires:
  emi_1525/1 -> cfblk66/1
  cfblk66/1 -> emi_1526/1

== system sampleModel646original/cfblk67 ==
  emi_534 : Inport
  Action Port : ActionPort  ActionPortLabel=else
  cfblk67 : Signum
  emi_535 : Outport
  wires:
  emi_534/1 -> cfblk67/1
  cfblk67/1 -> emi_535/1

== system sampleModel646original/cfblk69 ==
  emi_1252 : Inport
  Action Port : ActionPort  ActionPortLabel=else
  cfblk69 : Sqrt  SaturateOnIntegerOverflow=on
  emi_1253 : Outport
  wires:
  emi_1252/1 -> cfblk69/1
  cfblk69/1 -> emi_1253/1

== system sampleModel646original/cfblk71 ==
  emi_1778 : Inport
  Action Port : ActionPort  ActionPortLabel=else
  cfblk71 : ComplexToMagnitudeAngle
  emi_1779 : Outport
  emi_1780 : Outport  Port=2
  wires:
  emi_1778/1 -> cfblk71/1
  cfblk71/1 -> emi_1779/1
  cfblk71/2 -> emi_1780/1

== system sampleModel646original/cfblk73 ==
  emi_1698 : Inport
  Action Port : ActionPort  ActionPortLabel=else
  cfblk73 : Sqrt  SaturateOnIntegerOverflow=on
  emi_1699 : Outport
  wires:
  emi_1698/1 -> cfblk73/1
  cfblk73/1 -> emi_1699/1

== system sampleModel646original/cfblk77 ==
  emi_1840 : Inport
  Action Port : ActionPort  ActionPortLabel=else
  cfblk77 : UnaryMinus
  emi_1841 : Outport
  wires:
  emi_1840/1 -> cfblk77/1
  cfblk77/1 -> emi_1841/1

== system sampleModel646original/cfblk78 ==
  emi_1892 : Inport
  Action Port : ActionPort  ActionPortLabel=else
  cfblk78 : PermuteDimensions
  emi_1893 : Outport
  wires:
  emi_1892/1 -> cfblk78/1
  cfblk78/1 -> emi_1893/1

== system sampleModel646original/cfblk79 ==
  emi_1940 : Inport
  Action Port : ActionPort  ActionPortLabel=else
  cfblk79 : Sqrt  SaturateOnIntegerOverflow=on
  emi_1941 : Outport
  wires:
  emi_1940/1 -> cfblk79/1
  cfblk79/1 -> emi_1941/1

== system sampleModel646original/cfblk83 ==
  emi_2178 : Inport
  Action Port : ActionPort  ActionPortLabel=else
  cfblk83 : Subsystem
  emi_2179 : Outport
  wires:
  emi_2178/1 -> cfblk83/1(cfblk1)
  cfblk83/1(cfblk2) -> emi_2179/1

== system sampleModel646original/cfblk84 ==
  cfblk1 : Inport
  cfblk3 : slpidlib/PID Controller  Controller=PID  Form=Parallel  TimeDomain=Discrete-time  UseExternalTs=off  SampleTime=1  IntegratorMethod=Forward Euler  FilterMethod=Forward Euler  ControllerParametersSource=internal  P=1  I=1  D=0  UseFilter=on  N=100  TunerSelectOption=Transfer Function Based (PID Tuner App)  InitialConditionSource=internal  InitialConditionForIntegrator=0  InitialConditionForFilter=0  DifferentiatorICPrevScaledInput=0  ExternalReset=none  TrackingMode=off  Kt=1  LimitOutput=off  SatLimitsSource=internal  UpperSaturationLimit=inf  LowerSaturationLimit=-inf  LinearizeAsGain=off  AntiWindupMode=none  Kb=1  POutMin=[]  POutMax=[]  IOutMin=[]  IOutMax=[]  DOutMin=[]  DOutMax=[]  NOutMin=[]  NOutMax=[]  SumOutMin=[]  SumOutMax=[]  SaturationOutMin=[]  SaturationOutMax=[]  PParamMin=[]  PParamMax=[]  IParamMin=[]  IParamMax=[]  DParamMin=[]  DParamMax=[]  NParamMin=[]  NParamMax=[]  KbParamMin=[]  KbParamMax=[]  KtParamMin=[]  KtParamMax=[]  KbOutMin=[]  KbOutMax=[]  KtOutMin=[]  KtOutMax=[]  IntegratorOutMin=[]  IntegratorOutMax=[]  FilterOutMin=[]  FilterOutMax=[]  SumI1OutMin=[]  SumI1OutMax=[]  SumI2OutMin=[]  SumI2OutMax=[]  SumI3OutMin=[]  SumI3OutMax=[]  SumI4OutMin=[]  SumI4OutMax=[]  SumDOutMin=[]  SumDOutMax=[]  DifferentiatorOutMin=[]  DifferentiatorOutMax=[]  FilterDiffOutCoefMin=[]  FilterDiffOutCoefMax=[]  ReciprocalOutMin=[]  ReciprocalOutMax=[]  SumDenOutMin=[]  SumDenOutMax=[]  SumNumOutMin=[]  SumNumOutMax=[]  DivideOutMin=[]  DivideOutMax=[]  UdiffTsProdOutMin=[]  UdiffTsProdOutMax=[]  NTsProdOutMin=[]  NTsProdOutMax=[]  UintegralTsProdOutMin=[]  UintegralTsProdOutMax=[]  UngainTsProdOutMin=[]  UngainTsProdOutMax=[]  IntegratorContinuousStateAttributes=''  IntegratorStateMustResolveToSignalObject=off  IntegratorRTWStateStorageClass=Auto  FilterContinuousStateAttributes=''  FilterStateMustResolveToSignalObject=off  FilterRTWStateStorageClass=Auto  ParallelPVariant=InternalParameters  IdealPVariant=Disabled  IVariant=InternalParameters  DVariant=InternalParameters  IntegratorVariant=Discrete  SatVariant=Disabled  AWVariant=Passthrough  PCopyVariant=Disabled  TRVariant=Disabled  FdbkBlocksVariant=Forward  IdealPFdbkVariant=Disabled  SatFdbkVariant=Disabled  DerivativeFilterVariant=ForwardEulerFilter  NVariant=InternalParameters  NCopyVariant=Disabled  FilterICVariant=InternalICsFilter  IntegratorICVariant=InternalICs  ExternalResetVariant=Disabled  TRSumVariant=Passthrough  SumFdbkVariant=Disabled  SumVariant=Sum_PID  TsampFilterVariant=InternalTs  TsampNgainVariant=Passthrough  TsampIntegralVariant=Passthrough  ExternalSaturationOutDataTypeStr=Inherit: Same as second input
  cfblk4 : Sum  Inputs=+-
  cfblk5 : Trigonometry
  cfblk2 : Outport
  wires:
  cfblk5/1 -> cfblk2/1, cfblk4/2
  cfblk3/1 -> cfblk5/1
  cfblk1/1 -> cfblk3/1, cfblk4/1

== system sampleModel646original/cfblk85 ==
  cfblk1 : Inport
  cfblk3 : Gain  Gain=[-618223148.246293]
  cfblk4 : Sqrt  Operator=rSqrt  AlgorithmType=Newton-Raphson  SaturateOnIntegerOverflow=on
  cfblk5 : Signum
  cfblk2 : Outport
  wires:
  cfblk3/1 -> cfblk5/1
  cfblk4/1 -> cfblk3/1
  cfblk5/1 -> cfblk2/1
  cfblk1/1 -> cfblk4/1

== system sampleModel646original/cfblk86 ==
  cfblk1 : Inport
  cfblk3 : Gain  Gain=[-44772422.144375]
  cfblk4 : Product  Inputs=*
  cfblk5 : Sum  Inputs=+-
  cfblk2 : Outport
  wires:
  cfblk5/1 -> cfblk2/1
  cfblk4/1 -> cfblk5/1, cfblk5/2
  cfblk1/1 -> cfblk3/1
  cfblk3/1 -> cfblk4/1

== system sampleModel646original/cfblk87 ==
  cfblk1 : Inport
  cfblk3 : simulink/Discrete/Transfer Fcn Real Zero  ZeroZ=0.75  ICPrevInput=0.0  DoSatur=off
      settings: SourceProductBaseCode=SL
  cfblk4 : Reshape
  cfblk5 : Delay  SampleTime=1
  cfblk2 : Outport
  wires:
  cfblk3/1 -> cfblk4/1
  cfblk1/1 -> cfblk2/1
  cfblk4/1 -> cfblk5/1
  cfblk5/1 -> cfblk3/1

== system sampleModel646original/cfblk88 ==
  cfblk1 : Inport
  cfblk3 : Sin  TimeSource=Use external signal  SampleTime=0
  cfblk2 : Outport
  wires:
  cfblk1/1 -> cfblk2/1, cfblk3/1

== system sampleModel646original/cfblk89 ==
  cfblk1 : Inport
  cfblk3 : Math  Operator=pow  SaturateOnIntegerOverflow=on
  cfblk2 : Outport
  wires:
  cfblk1/1 -> cfblk3/1, cfblk3/2
  cfblk3/1 -> cfblk2/1

== system sampleModel646original/cfblk9 ==
  emi_2016 : Inport
  Action Port : ActionPort  ActionPortLabel=else
  cfblk9 : PermuteDimensions
  emi_2017 : Outport
  wires:
  emi_2016/1 -> cfblk9/1
  cfblk9/1 -> emi_2017/1

== system sampleModel646original/cfblk90 ==
  cfblk1 : Inport
  cfblk3 : ComplexToRealImag
  cfblk2 : Outport
  wires:
  cfblk3/1 -> cfblk2/1
  cfblk1/1 -> cfblk3/1

== system sampleModel646original/cfblk91 ==
  cfblk1 : Inport
  cfblk3 : Rounding
  cfblk2 : Outport
  wires:
  cfblk3/1 -> cfblk2/1
  cfblk1/1 -> cfblk3/1

== system sampleModel646original/cfblk92 ==
  cfblk1 : Inport
  cfblk3 : Assignment  DiagnosticForDimensions=Warning  IndexOptions=Index vector (dialog)  Indices=1  OutputSizes=1
  cfblk4 : Sum
  cfblk5 : Delay  SampleTime=1
  cfblk2 : Outport
  wires:
  cfblk4/1 -> cfblk3/1, cfblk3/2
  cfblk1/1 -> cfblk2/1, cfblk4/2
  cfblk3/1 -> cfblk5/1
  cfblk5/1 -> cfblk4/1

== system sampleModel646original/cfblk93 ==
  cfblk1 : Inport
  cfblk3 : Trigonometry
  cfblk2 : Outport
  wires:
  cfblk3/1 -> cfblk2/1
  cfblk1/1 -> cfblk3/1

== system sampleModel646original/cfblk96 ==
  cfblk1 : Inport
  Action Port : ActionPort  ActionPortLabel=if(u1 >= 0)
  cfblk3 : Product  Inputs=*
  cfblk4 : Trigonometry
  cfblk2 : Outport
  wires:
  cfblk1/1 -> cfblk4/1
  cfblk4/1 -> cfblk2/1, cfblk3/1

== system sampleModel646original/cfblk97 ==
  cfblk1 : Inport
  Action Port : ActionPort  ActionPortLabel=else
  cfblk3 : DiscreteStateSpace  SampleTime=-1
  cfblk4 : Squeeze
  cfblk5 : Delay
  cfblk2 : Outport
  wires:
  cfblk1/1 -> cfblk2/1
  cfblk3/1 -> cfblk4/1
  cfblk4/1 -> cfblk5/1
  cfblk5/1 -> cfblk3/1

== system sampleModel646original/cfblk98 ==
  cfblk1 : Inport
  Action Port : ActionPort  ActionPortLabel=if(u1 >= 0)
  cfblk3 : Math  Operator=square  SaturateOnIntegerOverflow=on
  cfblk2 : Outport
  wires:
  cfblk1/1 -> cfblk3/1
  cfblk3/1 -> cfblk2/1

== system sampleModel646original/cfblk99 ==
  cfblk1 : Inport
  Action Port : ActionPort  ActionPortLabel=else
  cfblk3 : Trigonometry
  cfblk2 : Outport
  wires:
  cfblk3/1 -> cfblk2/1
  cfblk1/1 -> cfblk3/1

== system sampleModel646original/emi_1017 ==
  In1 : Inport
  emi_1018 : Inport  Port=2
  emi_1020 : Quantizer
  emi_1021 : slpidlib/PID Controller  Controller=PID  Form=Parallel  TimeDomain=Discrete-time  UseExternalTs=off  SampleTime=-1  IntegratorMethod=Forward Euler  FilterMethod=Forward Euler  ControllerParametersSource=internal  P=1  I=1  D=0  UseFilter=on  N=100  TunerSelectOption=Transfer Function Based (PID Tuner App)  InitialConditionSource=internal  InitialConditionForIntegrator=0  InitialConditionForFilter=0  DifferentiatorICPrevScaledInput=0  ExternalReset=none  TrackingMode=off  Kt=1  LimitOutput=off  SatLimitsSource=internal  UpperSaturationLimit=inf  LowerSaturationLimit=-inf  LinearizeAsGain=off  AntiWindupMode=none  Kb=1  POutMin=[]  POutMax=[]  IOutMin=[]  IOutMax=[]  DOutMin=[]  DOutMax=[]  NOutMin=[]  NOutMax=[]  SumOutMin=[]  SumOutMax=[]  SaturationOutMin=[]  SaturationOutMax=[]  PParamMin=[]  PParamMax=[]  IParamMin=[]  IParamMax=[]  DParamMin=[]  DParamMax=[]  NParamMin=[]  NParamMax=[]  KbParamMin=[]  KbParamMax=[]  KtParamMin=[]  KtParamMax=[]  KbOutMin=[]  KbOutMax=[]  KtOutMin=[]  KtOutMax=[]  IntegratorOutMin=[]  IntegratorOutMax=[]  FilterOutMin=[]  FilterOutMax=[]  SumI1OutMin=[]  SumI1OutMax=[]  SumI2OutMin=[]  SumI2OutMax=[]  SumI3OutMin=[]  SumI3OutMax=[]  SumI4OutMin=[]  SumI4OutMax=[]  SumDOutMin=[]  SumDOutMax=[]  DifferentiatorOutMin=[]  DifferentiatorOutMax=[]  FilterDiffOutCoefMin=[]  FilterDiffOutCoefMax=[]  ReciprocalOutMin=[]  ReciprocalOutMax=[]  SumDenOutMin=[]  SumDenOutMax=[]  SumNumOutMin=[]  SumNumOutMax=[]  DivideOutMin=[]  DivideOutMax=[]  UdiffTsProdOutMin=[]  UdiffTsProdOutMax=[]  NTsProdOutMin=[]  NTsProdOutMax=[]  UintegralTsProdOutMin=[]  UintegralTsProdOutMax=[]  UngainTsProdOutMin=[]  UngainTsProdOutMax=[]  IntegratorContinuousStateAttributes=''  IntegratorStateMustResolveToSignalObject=off  IntegratorRTWStateStorageClass=Auto  FilterContinuousStateAttributes=''  FilterStateMustResolveToSignalObject=off  FilterRTWStateStorageClass=Auto  ParallelPVariant=InternalParameters  IdealPVariant=Disabled  IVariant=InternalParameters  DVariant=InternalParameters  IntegratorVariant=Discrete  SatVariant=Disabled  AWVariant=Passthrough  PCopyVariant=Disabled  TRVariant=Disabled  FdbkBlocksVariant=Forward  IdealPFdbkVariant=Disabled  SatFdbkVariant=Disabled  DerivativeFilterVariant=ForwardEulerFilter  NVariant=InternalParameters  NCopyVariant=Disabled  FilterICVariant=InternalICsFilter  IntegratorICVariant=InternalICs  ExternalResetVariant=Disabled  TRSumVariant=Passthrough  SumFdbkVariant=Disabled  SumVariant=Sum_PID  TsampFilterVariant=InternalTs  TsampNgainVariant=Passthrough  TsampIntegralVariant=Passthrough  ExternalSaturationOutDataTypeStr=Inherit: Same as second input
  emi_1022 : DiscreteFilter
  emi_1023 : Product  Inputs=*
  emi_1024 : simulink/Discontinuities/PWM  DisableCoverage=on  Period=1  DisallowZeroDutyCycle=off  RunAtFixedTimeIntervals=off  SampleTime=0.1
  emi_1025 : UnaryMinus
  emi_1026 : Math  SaturateOnIntegerOverflow=on
  emi_1027 : Sqrt  Operator=rSqrt  SaturateOnIntegerOverflow=on
  emi_1028 : DiscreteStateSpace  SampleTime=-1
  emi_1029 : simulink/Discrete/Discrete Derivative  gainval=1.0  ICPrevScaledInput=0.0  OutMin=[]  OutMax=[]  OutDataType=fixdt(1, 16)  OutScaling=2^-10  DoSatur=off
  emi_1030 : Quantizer
  emi_1031 : Trigonometry
  emi_1032 : Abs
  emi_1033 : RateLimiter  SampleTimeMode=inherited
  emi_1034 : DiscreteFir
  emi_1035 : RateLimiter  SampleTimeMode=inherited
  emi_1036 : simulink/Discrete/Difference  ICPrevInput=0.0  OutMin=[]  OutMax=[]  OutDataType=fixdt(1, 16)  OutScaling=2^-10  DoSatur=off
  emi_1037 : simulink/Discontinuities/PWM  DisableCoverage=on  Period=1  DisallowZeroDutyCycle=off  RunAtFixedTimeIntervals=off  SampleTime=0.1
  emi_1038 : Quantizer
  emi_1039 : simulink/Discontinuities/Wrap To Zero  Threshold=255
      settings: SourceProductBaseCode=SL
  emi_1040 : Abs
  emi_1041 : DiscreteFir
  emi_1042 : simulink/Discrete/Transfer Fcn First Order  PoleZ=0.95  ICPrevOutput=0.0  DoSatur=off
  emi_1043 : Sin  TimeSource=Use external signal  SampleTime=0
  emi_1044 : Sin  TimeSource=Use external signal  SampleTime=0
  emi_1045 : DeadZone  SaturateOnIntegerOverflow=on
  emi_1046 : Sqrt  Operator=rSqrt  SaturateOnIntegerOverflow=on
  emi_1047 : DeadZone  SaturateOnIntegerOverflow=on
  emi_1048 : simulink/Discontinuities/Wrap To Zero  Threshold=255
      settings: SourceProductBaseCode=SL
  emi_1049 : Sin  TimeSource=Use external signal  SampleTime=0
  emi_1050 : DiscreteFilter
  emi_1051 : MinMax
  emi_1052 : DiscreteFilter
  emi_1053 : RandomNumber  SampleTime=0.1
  Out1 : Outport
  emi_1019 : Outport  Port=2
  wires:
  In1/1 -> Out1/1
  emi_1020/1 -> emi_1021/1
  emi_1021/1 -> emi_1022/1
  emi_1022/1 -> emi_1023/1
  emi_1023/1 -> emi_1024/1
  emi_1024/1 -> emi_1025/1
  emi_1025/1 -> emi_1026/1
  emi_1026/1 -> emi_1027/1
  emi_1027/1 -> emi_1028/1
  emi_1028/1 -> emi_1029/1
  emi_1029/1 -> emi_1030/1
  emi_1030/1 -> emi_1031/1
  emi_1031/1 -> emi_1032/1
  emi_1032/1 -> emi_1033/1
  emi_1033/1 -> emi_1034/1
  emi_1034/1 -> emi_1035/1
  emi_1035/1 -> emi_1036/1
  emi_1036/1 -> emi_1037/1
  emi_1037/1 -> emi_1038/1
  emi_1038/1 -> emi_1039/1
  emi_1039/1 -> emi_1040/1
  emi_1040/1 -> emi_1041/1
  emi_1041/1 -> emi_1042/1
  emi_1042/1 -> emi_1043/1
  emi_1043/1 -> emi_1044/1
  emi_1044/1 -> emi_1045/1
  emi_1045/1 -> emi_1046/1
  emi_1046/1 -> emi_1047/1
  emi_1047/1 -> emi_1048/1
  emi_1048/1 -> emi_1049/1
  emi_1049/1 -> emi_1050/1
  emi_1050/1 -> emi_1051/1
  emi_1051/1 -> emi_1052/1
  emi_1053/1 -> emi_1020/1
  emi_1052/1 -> emi_1019/1

== system sampleModel646original/emi_1061 ==
  emi_1068 : Inport
  Action Port : ActionPort  ActionPortLabel=if(0 > u1)
  emi_{1065,1075,1083,1096} (4 alike) : MinMax
  emi_1066 : Trigonometry
  emi_{1067,1071,1085,1095} (4 alike) : Math  SaturateOnIntegerOverflow=on
  emi_1070 : Sum  Inputs=+
  emi_1072 : Sum  Inputs=+
  emi_1073 : Product  Inputs=*
  emi_1074 : Rounding
  emi_1076 : Sqrt  Operator=rSqrt  SaturateOnIntegerOverflow=on
  emi_1077 : Sum  Inputs=+
  emi_1078 : Sqrt  Operator=rSqrt  SaturateOnIntegerOverflow=on
  emi_1079 : Rounding
  emi_1080 : Trigonometry
  emi_1081 : Sqrt  Operator=rSqrt  SaturateOnIntegerOverflow=on
  emi_1082 : Product  Inputs=*
  emi_1084 : Rounding
  emi_1086 : Product  Inputs=*
  emi_1087 : Sin  TimeSource=Use external signal  SampleTime=0
  emi_1088 : Trigonometry
  emi_1089 : Gain
  emi_1090 : Abs
  emi_1091 : Gain
  emi_1092 : UnaryMinus
  emi_1093 : Abs
  emi_1094 : Abs
  emi_1097 : UnaryMinus
  emi_1098 : Ground
  emi_1069 : Outport
  wires:
  emi_1068/1 -> emi_1065/1
  emi_1065/1 -> emi_1066/1
  emi_1066/1 -> emi_1067/1
  emi_1070/1 -> emi_1071/1
  emi_1071/1 -> emi_1072/1
  emi_1072/1 -> emi_1073/1
  emi_1073/1 -> emi_1074/1
  emi_1074/1 -> emi_1075/1
  emi_1075/1 -> emi_1076/1
  emi_1076/1 -> emi_1077/1
  emi_1077/1 -> emi_1078/1
  emi_1078/1 -> emi_1079/1
  emi_1079/1 -> emi_1080/1
  emi_1080/1 -> emi_1081/1
  emi_1081/1 -> emi_1082/1
  emi_1082/1 -> emi_1083/1
  emi_1083/1 -> emi_1084/1
  emi_1084/1 -> emi_1085/1
  emi_1085/1 -> emi_1086/1
  emi_1086/1 -> emi_1087/1
  emi_1087/1 -> emi_1088/1
  emi_1088/1 -> emi_1089/1
  emi_1089/1 -> emi_1090/1
  emi_1090/1 -> emi_1091/1
  emi_1091/1 -> emi_1092/1
  emi_1092/1 -> emi_1093/1
  emi_1093/1 -> emi_1094/1
  emi_1094/1 -> emi_1095/1
  emi_1095/1 -> emi_1096/1
  emi_1096/1 -> emi_1097/1
  emi_1098/1 -> emi_1070/1
  emi_1097/1 -> emi_1069/1
